simulink model "sampleModel19"  (R2021b)
settings: Solver=VariableStepAuto  StartTime=0.0  StopTime=10.0  RelTol=1e-3
undefined symbols (not defined in the file or in its folder): DiscIntNeverNeededParam
libraries: simulink x12, slpidlib x1
settings Model: Creator=user  LastModifiedBy=user

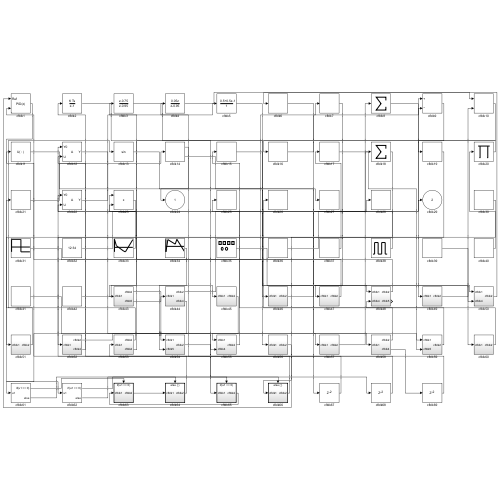
[thumbnail: Simulink's stored preview of the top-level diagram]
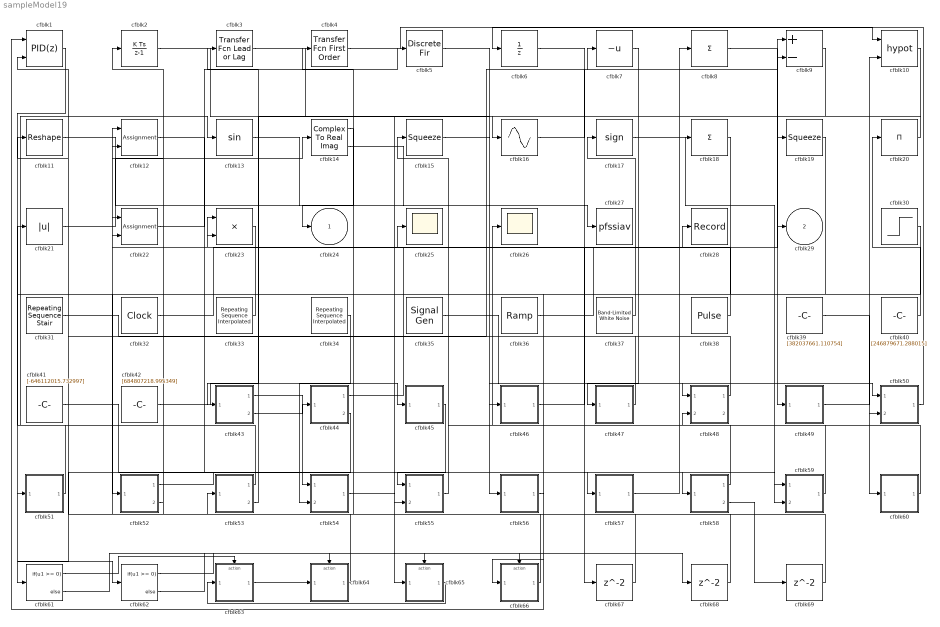
== system sampleModel19 ==
  cfblk1 : slpidlib/PID Controller (2DOF)  Controller=PID  Form=Parallel  TimeDomain=Discrete-time  UseExternalTs=off  SampleTime=1  IntegratorMethod=Forward Euler  FilterMethod=Forward Euler  ControllerParametersSource=internal  P=1  I=1  D=0  UseFilter=on  N=100  b=1  c=1  TunerSelectOption=Transfer Function Based (PID Tuner App)  InitialConditionSource=internal  InitialConditionForIntegrator=0  InitialConditionForFilter=0  DifferentiatorICPrevScaledInput=0  ExternalReset=none  TrackingMode=off  Kt=1  LimitOutput=off  SatLimitsSource=internal  UpperSaturationLimit=inf  LowerSaturationLimit=-inf  LinearizeAsGain=off  AntiWindupMode=none  Kb=1  POutMin=[]  POutMax=[]  IOutMin=[]  IOutMax=[]  DOutMin=[]  DOutMax=[]  NOutMin=[]  NOutMax=[]  bOutMin=[]  bOutMax=[]  cOutMin=[]  cOutMax=[]  SumOutMin=[]  SumOutMax=[]  SaturationOutMin=[]  SaturationOutMax=[]  PParamMin=[]  PParamMax=[]  IParamMin=[]  IParamMax=[]  DParamMin=[]  DParamMax=[]  NParamMin=[]  NParamMax=[]  bParamMin=[]  bParamMax=[]  cParamMin=[]  cParamMax=[]  KbParamMin=[]  KbParamMax=[]  KtParamMin=[]  KtParamMax=[]  KbOutMin=[]  KbOutMax=[]  KtOutMin=[]  KtOutMax=[]  IntegratorOutMin=[]  IntegratorOutMax=[]  FilterOutMin=[]  FilterOutMax=[]  SumI1OutMin=[]  SumI1OutMax=[]  SumI2OutMin=[]  SumI2OutMax=[]  SumI3OutMin=[]  SumI3OutMax=[]  SumI4OutMin=[]  SumI4OutMax=[]  SumDOutMin=[]  SumDOutMax=[]  Sum1OutMin=[]  Sum1OutMax=[]  Sum2OutMin=[]  Sum2OutMax=[]  Sum3OutMin=[]  Sum3OutMax=[]  DifferentiatorOutMin=[]  DifferentiatorOutMax=[]  FilterDiffOutCoefMin=[]  FilterDiffOutCoefMax=[]  ReciprocalOutMin=[]  ReciprocalOutMax=[]  SumDenOutMin=[]  SumDenOutMax=[]  SumNumOutMin=[]  SumNumOutMax=[]  DivideOutMin=[]  DivideOutMax=[]  UdiffTsProdOutMin=[]  UdiffTsProdOutMax=[]  NTsProdOutMin=[]  NTsProdOutMax=[]  UintegralTsProdOutMin=[]  UintegralTsProdOutMax=[]  UngainTsProdOutMin=[]  UngainTsProdOutMax=[]  IntegratorContinuousStateAttributes=''  IntegratorStateMustResolveToSignalObject=off  IntegratorRTWStateStorageClass=Auto  FilterContinuousStateAttributes=''  FilterStateMustResolveToSignalObject=off  FilterRTWStateStorageClass=Auto  ParallelPVariant=InternalParameters  IdealPVariant=Disabled  IVariant=InternalParameters  DVariant=InternalParameters  bVariant=InternalParameters  cVariant=InternalParameters  IntegratorVariant=Discrete  SatVariant=Disabled  AWVariant=Passthrough  PCopyVariant=Disabled  TRVariant=Disabled  FdbkBlocksVariant=Forward  IdealPFdbkVariant=Disabled  SatFdbkVariant=Disabled  DerivativeFilterVariant=ForwardEulerFilter  NVariant=InternalParameters  NCopyVariant=Disabled  FilterICVariant=InternalICsFilter  IntegratorICVariant=InternalICs  ExternalResetVariant=Disabled  TRSumVariant=Passthrough  SumFdbkVariant=Disabled  SumVariant=Sum_PID  TsampFilterVariant=InternalTs  TsampNgainVariant=Passthrough  TsampIntegralVariant=Passthrough  ExternalSaturationOutDataTypeStr=Inherit: Same as second input
      settings: SourceProductBaseCode=SL
  cfblk10 : Math  Operator=hypot  SaturateOnIntegerOverflow=on
  cfblk11 : Reshape
  cfblk12 : Assignment  DiagnosticForDimensions=Warning  IndexOptions=Index vector (dialog)  Indices=1  OutputSizes=1
  cfblk13 : Trigonometry
  cfblk14 : ComplexToRealImag
  cfblk15 : Squeeze
  cfblk16 : Sin  TimeSource=Use external signal  SampleTime=0
  cfblk17 : Signum
  cfblk18 : Sum  Inputs=+
  cfblk19 : Squeeze
  cfblk2 : DiscreteIntegrator  ICPrevOutput=DiscIntNeverNeededParam  ICPrevScaledInput=DiscIntNeverNeededParam
  cfblk20 : Product  Inputs=*
  cfblk21 : Abs
  cfblk22 : Assignment  DiagnosticForDimensions=Warning  IndexOptions=Index vector (dialog)  Indices=1  OutputSizes=1
  cfblk23 : Product
  cfblk25 : Scope
  cfblk26 : Scope
  cfblk27 : ToWorkspace  VariableName=pfssiav  SaveFormat=Timeseries  SampleTime=-1
  cfblk28 : Record  FileSettingsInternal="{\"entries\":[{\"content\":{\"excelSettings\":{\"content\":{},\"type\":\"Streamout.ExcelSettings\"}},\"type\":\"Streamout.FileSettingStorage\",\"uuid\":\"f226d651-ed76-4685-bd0d-a7206099ba54\"}],\"packageUris\":[\"http://schema.mathworks.com/mf0/streamout_blocks/R2020a\"],\"version\":\"1.0\"}"  SignalsInternal="{\"entries\":[{\"content\":{\"signals\":[{\"content\":{\"blockPath\":[\"sampleModel19/cfblk28\"],\"channel\":[],\"dimensions\":[1],\"domain\":\"sampleModel19/cfblk28\",\"lineColor\":\"#b746ff\",\"plots\":[1],\"port\":1,\"sid\":[\"\"],\"signalID\":797,\"signalName\":\"cfblk46\"},\"type\":\"RecordBlkView.Signal\",\"uuid\":\"ee6bbbbf-7b49-4810-a904-b0b81152954a\"}]},\"type\":\"RecordBlkView.InputSignals\",\"uuid\":\"19e5beda-3c9f-445c-ba6f-61ea0a1a64e1\"}],\"packageUris\":[\"http://schema.mathworks.com/mf0/streamout_blocks/R2020a\"],\"version\":\"1.0\"}"  VisualizationBindings="{\"sparklinesplugin\":{\"info\":[{\"bindingParametersList\":[],\"subplotID\":1}]}}"
  cfblk3 : simulink/Discrete/Transfer Fcn Lead or Lag  PoleZ=0.95  ZeroZ=0.75  ICPrevOutput=0.0  ICPrevInput=0.0  DoSatur=off
      settings: SourceProductBaseCode=SL
  cfblk30 : Step  Time=[38.000000]  Before=[19293273.623970]  After=[413926557.525764]  SampleTime=0
  cfblk31 : simulink/Sources/Repeating Sequence Stair  OutValues=[582347814.794268, -338661963.550210]  tsamp=-1  OutMin=[]  OutMax=[]  OutDataTypeStr=double  OutputDataTypeScalingMode=double  OutDataType=fixdt(0,8)  ConRadixGroup=Best Precision: Vector-wise  OutScaling=2^-12
  cfblk32 : DigitalClock
  cfblk33 : simulink/Sources/Repeating Sequence Interpolated  OutValues=[827350283.908176, 153409925.635676, -424181451.709205, -466270279.479304, 780356358.093050]  TimeValues=[0 0.1 0.5 0.6 1].'  LookUpMeth=Use Input Nearest  tsamp=0.01  OutMin=[]  OutMax=[]  OutDataTypeStr=double  OutputDataTypeScalingMode=double  OutDataType=fixdt(0,8)  OutScaling=2^-10
  cfblk34 : simulink/Sources/Repeating Sequence Interpolated  OutValues=[-699969224.824603, 892655139.539717, 301670629.198861, 964429137.746531, -612332611.980431]  TimeValues=[0 0.1 0.5 0.6 1].'  LookUpMeth=Use Input Above  tsamp=0.01  OutMin=[]  OutMax=[]  OutDataTypeStr=double  OutputDataTypeScalingMode=double  OutDataType=fixdt(0,8)  OutScaling=2^-10
  cfblk35 : SignalGenerator  WaveForm=square  Amplitude=[-12395821.292946]  Units=rad/sec
  cfblk36 : simulink/Sources/Ramp  slope=[1289.163040]  start=[32.043671]  InitialOutput=[-3800.474352]
  cfblk37 : simulink/Sources/Band-Limited White Noise  Cov=[596236290.793144]  Ts=0.1  seed=[5151631842.000000]
  cfblk38 : DiscretePulseGenerator  PulseType=Time based  Amplitude=[-893610121.964039]  Period=[84363192.211661]  PulseWidth=5  PhaseDelay=[6.000000]
  cfblk39 : Constant  Value=[382037661.110754]  SampleTime=1
  cfblk4 : simulink/Discrete/Transfer Fcn First Order  PoleZ=0.95  ICPrevOutput=0.0  DoSatur=off
  cfblk40 : Constant  Value=[246879671.288015]  SampleTime=1
  cfblk41 : Constant  Value=[-646112015.732997]  SampleTime=1
  cfblk42 : Constant  Value=[684807218.995349]  SampleTime=1
  cfblk43 : Subsystem
  cfblk44 : Subsystem
  cfblk45 : Subsystem
  cfblk46 : Subsystem
  cfblk47 : Subsystem
  cfblk48 : Subsystem
  cfblk49 : Subsystem
  cfblk5 : DiscreteFir  SampleTime=1
  cfblk50 : Subsystem
  cfblk51 : Subsystem
  cfblk52 : Subsystem
  cfblk53 : Subsystem
  cfblk54 : Subsystem
  cfblk55 : Subsystem
  cfblk56 : Subsystem
  cfblk57 : Subsystem
  cfblk58 : Subsystem
  cfblk59 : Subsystem
  cfblk6 : UnitDelay  HasFrameUpgradeWarning=on
  cfblk60 : Subsystem
  cfblk61 : If  IfExpression=u1 >= 0  SampleTime=1
  cfblk62 : If  IfExpression=u1 >= 0  SampleTime=1
  cfblk63 : Subsystem  TreatAsAtomicUnit=on
  cfblk64 : Subsystem  TreatAsAtomicUnit=on
  cfblk65 : Subsystem  TreatAsAtomicUnit=on
  cfblk66 : Subsystem  TreatAsAtomicUnit=on
  cfblk67 : Delay  SampleTime=1
  cfblk68 : Delay  SampleTime=1
  cfblk69 : Delay  SampleTime=1
  cfblk7 : UnaryMinus
  cfblk8 : Sum  Inputs=+
  cfblk9 : Sum  Inputs=+-
  cfblk24 : Outport
  cfblk29 : Outport  Port=2
  wires:
  cfblk21/1 -> cfblk14/1
  cfblk51/1(cfblk2) -> cfblk13/1
  cfblk33/1 -> cfblk12/1
  cfblk20/1 -> cfblk16/1
  cfblk1/1 -> cfblk62/1
  cfblk31/1 -> cfblk7/1
  cfblk12/1 -> cfblk58/1(cfblk1)
  cfblk65/1(cfblk2) -> cfblk63/1(cfblk1)
  cfblk66/1(cfblk2) -> cfblk22/1
  cfblk50/1(cfblk2) -> cfblk6/1
  cfblk42/1 -> cfblk45/1(cfblk1)
  cfblk13/1 -> cfblk27/1
  cfblk44/1(cfblk2) -> cfblk9/1
  cfblk45/1(cfblk2) -> cfblk55/1(cfblk1)
  cfblk60/1(cfblk2) -> cfblk26/1
  cfblk11/1 -> cfblk46/1(cfblk1)
  cfblk18/1 -> cfblk51/1(cfblk1)
  cfblk64/1(cfblk2) -> cfblk53/1(cfblk1)
  cfblk58/1(cfblk2) -> cfblk15/1
  cfblk5/1 -> cfblk50/1(cfblk1)
  cfblk55/1(cfblk2) -> cfblk25/1
  cfblk2/1 -> cfblk56/1(cfblk1)
  cfblk43/1(cfblk2) -> cfblk54/1(cfblk1)
  cfblk39/1 -> cfblk60/1(cfblk1)
  cfblk7/1 -> cfblk47/1(cfblk1)
  cfblk4/1 -> cfblk10/1
  cfblk23/1 -> cfblk22/2
  cfblk37/1 -> cfblk17/1
  cfblk57/1(cfblk2) -> cfblk8/1
  cfblk41/1 -> cfblk65/1(cfblk1)
  cfblk56/1(cfblk2) -> cfblk1/1
  cfblk8/1 -> cfblk49/1(cfblk1)
  cfblk19/1 -> cfblk66/1(cfblk1)
  cfblk34/1 -> cfblk54/2(cfblk5)
  cfblk36/1 -> cfblk29/1
  cfblk14/1 -> cfblk24/1
  cfblk10/1 -> cfblk43/1(cfblk1)
  cfblk40/1 -> cfblk20/1
  cfblk53/1(cfblk2) -> cfblk21/1
  cfblk63/1(cfblk2) -> cfblk64/1(cfblk1)
  cfblk15/1 -> cfblk50/2(cfblk4)
  cfblk46/1(cfblk2) -> cfblk28/1
  cfblk47/1(cfblk2) -> cfblk11/1
  cfblk17/1 -> cfblk59/1(cfblk1)
  cfblk16/1 -> cfblk9/2
  cfblk53/2(cfblk4) -> cfblk23/1
  cfblk49/1(cfblk2) -> cfblk10/2
  cfblk38/1 -> cfblk23/2
  cfblk44/2(cfblk4) -> cfblk61/1
  cfblk6/1 -> cfblk59/2(cfblk5)
  cfblk3/1 -> cfblk55/2(cfblk4)
  cfblk48/1(cfblk2) -> cfblk3/1
  cfblk32/1 -> cfblk18/1
  cfblk30/1 -> cfblk52/1(cfblk1)
  cfblk43/2(cfblk5) -> cfblk44/1(cfblk1)
  cfblk9/1 -> cfblk19/1
  cfblk22/1 -> cfblk5/1
  cfblk35/1 -> cfblk48/1(cfblk1)
  cfblk59/1(cfblk2) -> cfblk48/2(cfblk4)
  cfblk52/1(cfblk2) -> cfblk57/1(cfblk1)
  cfblk52/2(cfblk4) -> cfblk2/1
  cfblk61/1 -> cfblk63/Action
  cfblk61/2 -> cfblk64/Action
  cfblk62/1 -> cfblk65/Action
  cfblk62/2 -> cfblk66/Action
  cfblk14/2 -> cfblk67/1
  cfblk67/1 -> cfblk1/2
  cfblk54/1(cfblk2) -> cfblk68/1
  cfblk68/1 -> cfblk4/1
  cfblk58/2(cfblk4) -> cfblk69/1
  cfblk69/1 -> cfblk12/2

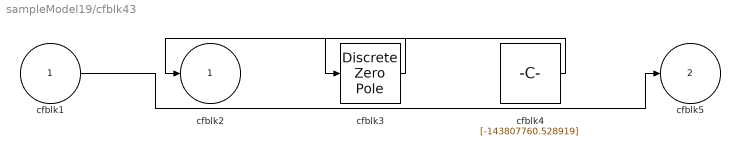
== system sampleModel19/cfblk43 ==
  cfblk1 : Inport
  cfblk3 : DiscreteZeroPole  Poles=[0 0.5]  Gain=1
  cfblk4 : Constant  Value=[-143807760.528919]  SampleTime=1
  cfblk2 : Outport
  cfblk5 : Outport  Port=2
  wires:
  cfblk3/1 -> cfblk2/1
  cfblk1/1 -> cfblk5/1
  cfblk4/1 -> cfblk3/1

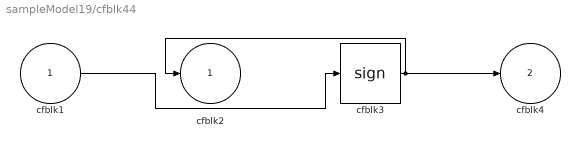
== system sampleModel19/cfblk44 ==
  cfblk1 : Inport
  cfblk3 : Signum
  cfblk2 : Outport
  cfblk4 : Outport  Port=2
  wires:
  cfblk3/1 -> cfblk2/1, cfblk4/1
  cfblk1/1 -> cfblk3/1

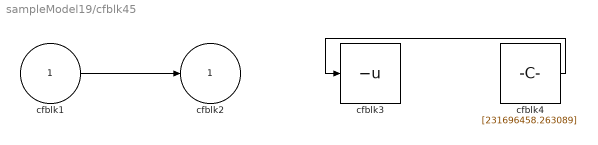
== system sampleModel19/cfblk45 ==
  cfblk1 : Inport
  cfblk3 : UnaryMinus
  cfblk4 : Constant  Value=[231696458.263089]  SampleTime=1
  cfblk2 : Outport
  wires:
  cfblk4/1 -> cfblk3/1
  cfblk1/1 -> cfblk2/1

== system sampleModel19/cfblk46 ==
  cfblk1 : Inport
  cfblk3 : Product  Inputs=*
  cfblk2 : Outport
  wires:
  cfblk3/1 -> cfblk2/1
  cfblk1/1 -> cfblk3/1

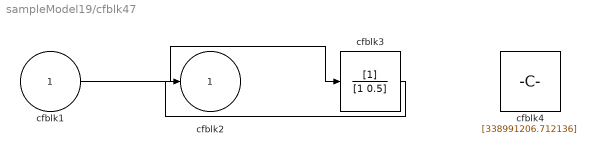
== system sampleModel19/cfblk47 ==
  cfblk1 : Inport
  cfblk3 : DiscreteFilter  SampleTime=1
  cfblk4 : Constant  Value=[338991206.712136]  SampleTime=1
  cfblk2 : Outport
  wires:
  cfblk1/1 -> cfblk3/1
  cfblk3/1 -> cfblk2/1

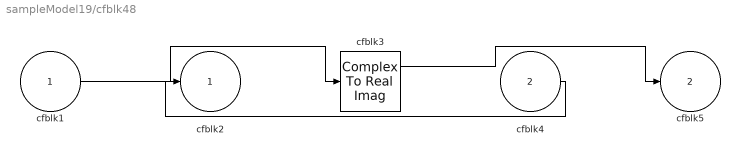
== system sampleModel19/cfblk48 ==
  cfblk1 : Inport
  cfblk4 : Inport  Port=2
  cfblk3 : ComplexToRealImag
  cfblk2 : Outport
  cfblk5 : Outport  Port=2
  wires:
  cfblk1/1 -> cfblk3/1
  cfblk4/1 -> cfblk2/1
  cfblk3/1 -> cfblk5/1

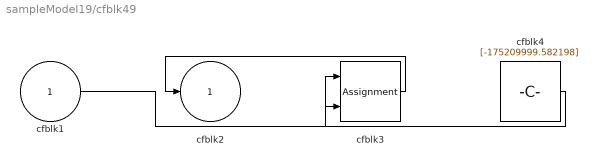
== system sampleModel19/cfblk49 ==
  cfblk1 : Inport
  cfblk3 : Assignment  DiagnosticForDimensions=Warning  IndexOptions=Index vector (dialog)  Indices=1  OutputSizes=1
  cfblk4 : Constant  Value=[-175209999.582198]  SampleTime=1
  cfblk2 : Outport
  wires:
  cfblk3/1 -> cfblk2/1
  cfblk1/1 -> cfblk3/1
  cfblk4/1 -> cfblk3/2

== system sampleModel19/cfblk50 ==
  cfblk1 : Inport
  cfblk4 : Inport  Port=2
  cfblk3 : PermuteDimensions
  cfblk2 : Outport
  wires:
  cfblk1/1 -> cfblk3/1
  cfblk4/1 -> cfblk2/1

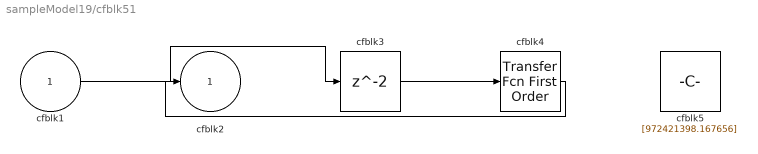
== system sampleModel19/cfblk51 ==
  cfblk1 : Inport
  cfblk3 : Delay  SampleTime=1
  cfblk4 : simulink/Discrete/Transfer Fcn First Order  PoleZ=0.95  ICPrevOutput=0.0  DoSatur=off
  cfblk5 : Constant  Value=[972421398.167656]  SampleTime=1
  cfblk2 : Outport
  wires:
  cfblk1/1 -> cfblk3/1
  cfblk4/1 -> cfblk2/1
  cfblk3/1 -> cfblk4/1

== system sampleModel19/cfblk52 ==
  cfblk1 : Inport
  cfblk3 : simulink/Discrete/Difference  ICPrevInput=0.0  OutMin=[]  OutMax=[]  OutDataTypeStr=Inherit: Inherit via back propagation  OutDataType=fixdt(1, 16)  OutScaling=2^-10  DoSatur=off
  cfblk2 : Outport
  cfblk4 : Outport  Port=2
  wires:
  cfblk1/1 -> cfblk3/1, cfblk2/1
  cfblk3/1 -> cfblk4/1

== system sampleModel19/cfblk53 ==
  cfblk1 : Inport
  cfblk3 : Squeeze
  cfblk2 : Outport
  cfblk4 : Outport  Port=2
  wires:
  cfblk1/1 -> cfblk4/1, cfblk3/1
  cfblk3/1 -> cfblk2/1

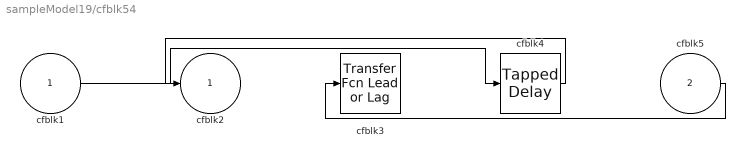
== system sampleModel19/cfblk54 ==
  cfblk1 : Inport
  cfblk5 : Inport  Port=2
  cfblk3 : simulink/Discrete/Transfer Fcn Lead or Lag  PoleZ=0.95  ZeroZ=0.75  ICPrevOutput=0.0  ICPrevInput=0.0  DoSatur=off
      settings: SourceProductBaseCode=SL
  cfblk4 : simulink/Discrete/Tapped Delay  vinit=0.0  samptime=-1  NumDelays=1  DelayOrder=Oldest  includeCurrent=off
  cfblk2 : Outport
  wires:
  cfblk1/1 -> cfblk4/1
  cfblk5/1 -> cfblk3/1
  cfblk4/1 -> cfblk2/1

== system sampleModel19/cfblk55 ==
  cfblk1 : Inport
  cfblk4 : Inport  Port=2
  cfblk3 : DiscreteStateSpace
  cfblk2 : Outport
  wires:
  cfblk3/1 -> cfblk2/1
  cfblk4/1 -> cfblk3/1

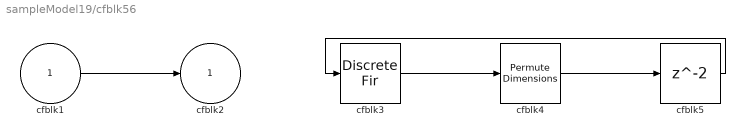
== system sampleModel19/cfblk56 ==
  cfblk1 : Inport
  cfblk3 : DiscreteFir  SampleTime=1
  cfblk4 : PermuteDimensions
  cfblk5 : Delay  SampleTime=1
  cfblk2 : Outport
  wires:
  cfblk1/1 -> cfblk2/1
  cfblk3/1 -> cfblk4/1
  cfblk4/1 -> cfblk5/1
  cfblk5/1 -> cfblk3/1

== system sampleModel19/cfblk57 ==
  cfblk1 : Inport
  cfblk3 : DiscreteIntegrator  ICPrevOutput=DiscIntNeverNeededParam  ICPrevScaledInput=DiscIntNeverNeededParam
  cfblk2 : Outport
  wires:
  cfblk3/1 -> cfblk2/1
  cfblk1/1 -> cfblk3/1

== system sampleModel19/cfblk58 ==
  cfblk1 : Inport
  cfblk3 : DiscreteIntegrator  ICPrevOutput=DiscIntNeverNeededParam  ICPrevScaledInput=DiscIntNeverNeededParam
  cfblk2 : Outport
  cfblk4 : Outport  Port=2
  wires:
  cfblk1/1 -> cfblk2/1, cfblk3/1
  cfblk3/1 -> cfblk4/1

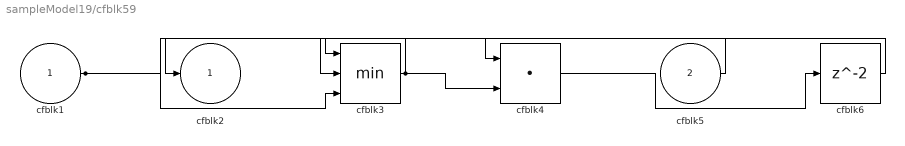
== system sampleModel19/cfblk59 ==
  cfblk1 : Inport
  cfblk5 : Inport  Port=2
  cfblk3 : MinMax  Inputs=3
  cfblk4 : DotProduct  InputSameDT=on  OutDataTypeStr=Inherit: Inherit via internal rule
  cfblk6 : Delay  SampleTime=1
  cfblk2 : Outport
  wires:
  cfblk5/1 -> cfblk4/1
  cfblk3/1 -> cfblk2/1, cfblk4/2
  cfblk1/1 -> cfblk3/2, cfblk3/3
  cfblk4/1 -> cfblk6/1
  cfblk6/1 -> cfblk3/1

== system sampleModel19/cfblk60 ==
  cfblk1 : Inport
  cfblk3 : Constant  Value=[-132616735.512844]  SampleTime=1
  cfblk2 : Outport
  wires:
  cfblk3/1 -> cfblk2/1

== system sampleModel19/cfblk63 ==
  cfblk1 : Inport
  Action Port : ActionPort  ActionPortLabel=if(u1 >= 0)
  cfblk3 : Delay  ShowEnablePort=on
      settings: InputPortMap=u0,e6
  cfblk2 : Outport
  wires:
  cfblk1/1 -> cfblk2/1, cfblk3/1, cfblk3/2

== system sampleModel19/cfblk64 ==
  cfblk1 : Inport
  Action Port : ActionPort  ActionPortLabel=else
  cfblk3 : ComplexToRealImag
  cfblk2 : Outport
  wires:
  cfblk1/1 -> cfblk3/1
  cfblk3/1 -> cfblk2/1

== system sampleModel19/cfblk65 ==
  cfblk1 : Inport
  Action Port : ActionPort  ActionPortLabel=if(u1 >= 0)
  cfblk3 : Squeeze
  cfblk2 : Outport
  wires:
  cfblk3/1 -> cfblk2/1
  cfblk1/1 -> cfblk3/1

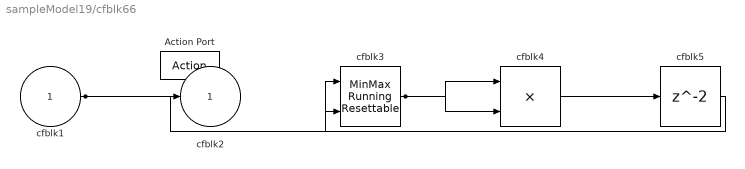
== system sampleModel19/cfblk66 ==
  cfblk1 : Inport
  Action Port : ActionPort  ActionPortLabel=else
  cfblk3 : simulink/Math Operations/MinMax Running Resettable  Function=min  vinit=0.0
  cfblk4 : Product  Inputs=**
  cfblk5 : Delay
  cfblk2 : Outport
  wires:
  cfblk1/1 -> cfblk3/1, cfblk2/1
  cfblk3/1 -> cfblk4/1, cfblk4/2
  cfblk4/1 -> cfblk5/1
  cfblk5/1 -> cfblk3/2
